simulink model "rotate_pid"  (R2021a)
settings: Solver=FixedStepDiscrete  StartTime=0.0  StopTime=5  FixedStep=0.01  RelTol=1e-3
values from neighbouring files (symbols this model uses):
  ticksPerRot = 20    [robotParameters.m]
  wheelR = 0.031    [robotParameters.m]
undefined symbols (not defined in the file or in its folder): InputPWM, WheelSpeed
libraries: mobileRoboticsTrainingLib x5, pid_lib x1
settings Model: EnablePacing=on  Creator=Boitumelo  LastModifiedBy=markl

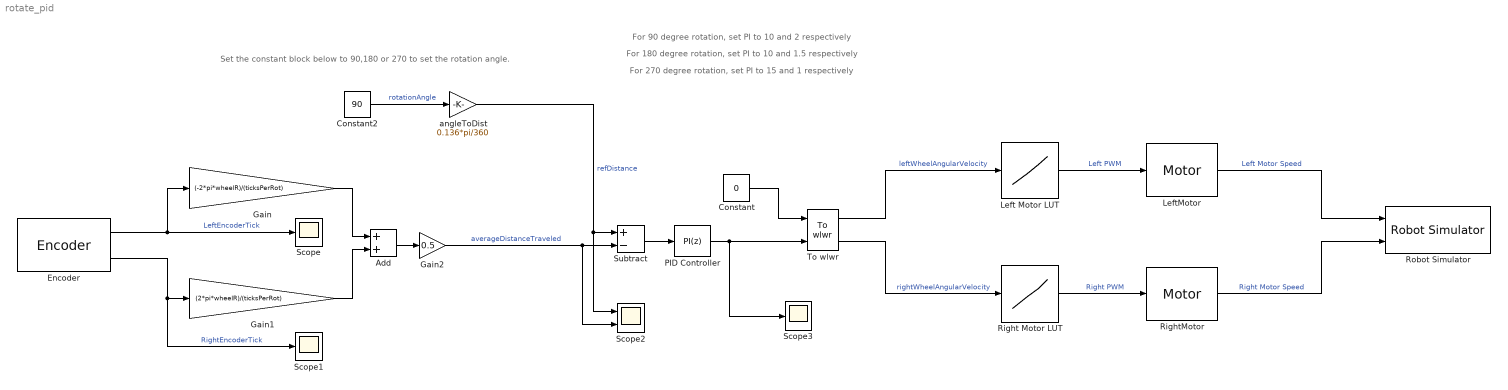
== system rotate_pid ==
  note: For 90 degree rotation, set PI to 10 and 2 respectively
  note: Set the constant block below to 90,180 or 270 to set the rotation angle.
  note: For 180 degree rotation, set PI to 10 and 1.5 respectively
  note: For 270 degree rotation, set PI to 15 and 1 respectively
  Add : Sum
  Constant : Constant  Value=0
  Constant2 : Constant  Value=90
  Encoder : mobileRoboticsTrainingLib/Encoder  axleLength=axleLength  wheelR=wheelR  ticksPerRot=ticksPerRot
      settings: SourceProductName=Mobile Robotics Training Library
  Gain : Gain  Gain=(-2*pi*wheelR)/(ticksPerRot)
  Gain1 : Gain  Gain=(2*pi*wheelR)/(ticksPerRot)
  Gain2 : Gain  Gain=0.5
  Left Motor LUT : Lookup_n-D  NumberOfTableDimensions=1  BreakpointsForDimension1=WheelSpeed  Table=InputPWM  InterpMethod=Nearest  ExtrapMethod=Clip  InternalRulePriority=Speed  RndMeth=Simplest  InputSameDT=on
  LeftMotor : mobileRoboticsTrainingLib/Motor  motorPlant=wheelMotorModel  sensorType=Speed
      settings: SourceProductName=Mobile Robotics Training Library
  PID Controller : pid_lib/PID Controller  Controller=PI  Form=Parallel  TimeDomain=Discrete-time  UseExternalTs=off  SampleTime=-1  IntegratorMethod=Forward Euler  FilterMethod=Forward Euler  ControllerParametersSource=internal  P=10  I=2  D=0.1  UseFilter=on  N=100  TunerSelectOption=Transfer Function Based (PID Tuner App)  InitialConditionSource=internal  InitialConditionForIntegrator=0  InitialConditionForFilter=0  DifferentiatorICPrevScaledInput=0  ExternalReset=none  TrackingMode=off  Kt=1  LimitOutput=on  SatLimitsSource=internal  UpperSaturationLimit=12.5106  LowerSaturationLimit=-12.5106  LinearizeAsGain=on  AntiWindupMode=clamping  Kb=1  POutMin=[]  POutMax=[]  IOutMin=[]  IOutMax=[]  DOutMin=[]  DOutMax=[]  NOutMin=[]  NOutMax=[]  SumOutMin=[]  SumOutMax=[]  SaturationOutMin=[]  SaturationOutMax=[]  PParamMin=[]  PParamMax=[]  IParamMin=[]  IParamMax=[]  DParamMin=[]  DParamMax=[]  NParamMin=[]  NParamMax=[]  KbParamMin=[]  KbParamMax=[]  KtParamMin=[]  KtParamMax=[]  KbOutMin=[]  KbOutMax=[]  KtOutMin=[]  KtOutMax=[]  IntegratorOutMin=[]  IntegratorOutMax=[]  FilterOutMin=[]  FilterOutMax=[]  SumI1OutMin=[]  SumI1OutMax=[]  SumI2OutMin=[]  SumI2OutMax=[]  SumI3OutMin=[]  SumI3OutMax=[]  SumI4OutMin=[]  SumI4OutMax=[]  SumDOutMin=[]  SumDOutMax=[]  DifferentiatorOutMin=[]  DifferentiatorOutMax=[]  FilterDiffOutCoefMin=[]  FilterDiffOutCoefMax=[]  ReciprocalOutMin=[]  ReciprocalOutMax=[]  SumDenOutMin=[]  SumDenOutMax=[]  SumNumOutMin=[]  SumNumOutMax=[]  DivideOutMin=[]  DivideOutMax=[]  UdiffTsProdOutMin=[]  UdiffTsProdOutMax=[]  NTsProdOutMin=[]  NTsProdOutMax=[]  UintegralTsProdOutMin=[]  UintegralTsProdOutMax=[]  UngainTsProdOutMin=[]  UngainTsProdOutMax=[]  IntegratorContinuousStateAttributes=''  IntegratorStateMustResolveToSignalObject=off  IntegratorRTWStateStorageClass=Auto  FilterContinuousStateAttributes=''  FilterStateMustResolveToSignalObject=off  FilterRTWStateStorageClass=Auto  ParallelPVariant=InternalParameters  IdealPVariant=Disabled  IVariant=InternalParameters  DVariant=Disabled  IntegratorVariant=Discrete  SatVariant=Enabled  AWVariant=DiscClampingParallel  PCopyVariant=Disabled  TRVariant=Disabled  FdbkBlocksVariant=Forward  IdealPFdbkVariant=Disabled  SatFdbkVariant=Disabled  DerivativeFilterVariant=Disabled  NVariant=Disabled  NCopyVariant=Disabled_SignalSpec  FilterICVariant=Disabled  IntegratorICVariant=InternalICs  ExternalResetVariant=Disabled  TRSumVariant=Passthrough  SumFdbkVariant=Disabled  SumVariant=Sum_PI  TsampFilterVariant=InternalTs  TsampNgainVariant=Passthrough  TsampIntegralVariant=Passthrough  ExternalSaturationOutDataTypeStr=Inherit: Same as second input  InitialConditionSetting=Output
  Right Motor LUT : Lookup_n-D  NumberOfTableDimensions=1  BreakpointsForDimension1=WheelSpeed  Table=InputPWM  InterpMethod=Nearest  ExtrapMethod=Clip  InternalRulePriority=Speed  RndMeth=Simplest  InputSameDT=on
  RightMotor : mobileRoboticsTrainingLib/Motor  motorPlant=wheelMotorModel  sensorType=Speed
      settings: SourceProductName=Mobile Robotics Training Library
  Robot Simulator : mobileRoboticsTrainingLib/Robot Simulator  Priority=99  mapVar=[]  startX=1  startY=1  startTheta=0  axleLength=axleLength  wheelR=wheelR
  Scope : Scope
  Scope1 : Scope
  Scope2 : Scope  NumInputPorts=2
  Scope3 : Scope
  Subtract : Sum  Inputs=+-
  To wlwr : mobileRoboticsTrainingLib/To wlwr  axleLength=axleLength  wheelR=wheelR
  angleToDist : Gain  Gain=0.136*pi/360
  wires:
  LeftMotor/1 -> Robot Simulator/1  "Left Motor Speed"
  RightMotor/1 -> Robot Simulator/2  "Right Motor Speed"
  Right Motor LUT/1 -> RightMotor/1  "Right PWM"
  Left Motor LUT/1 -> LeftMotor/1  "Left PWM"
  Encoder/1 -> Gain/1, Scope/1  "LeftEncoderTick"
  To wlwr/1 -> Left Motor LUT/1  "leftWheelAngularVelocity"
  To wlwr/2 -> Right Motor LUT/1  "rightWheelAngularVelocity"
  Encoder/2 -> Scope1/1, Gain1/1  "RightEncoderTick"
  Gain/1 -> Add/1
  Gain1/1 -> Add/2
  Add/1 -> Gain2/1
  Gain2/1 -> Subtract/2, Scope2/2  "averageDistanceTraveled"
  PID Controller/1 -> To wlwr/2, Scope3/1
  Constant/1 -> To wlwr/1
  angleToDist/1 -> Scope2/1, Subtract/1  "refDistance"
  Subtract/1 -> PID Controller/1
  Constant2/1 -> angleToDist/1  "rotationAngle"
